simulink library "Thermal_Node"  (R2018b)
settings: Solver=ode45  StartTime=0.0  StopTime=10.0  RelTol=1e-3  EnableMultiTasking=on
settings Model: Creator=Hafner  LastModifiedBy=drhf
settings DataIOCC: LimitDataPoints=on  SaveFormat=Array  SignalLoggingSaveFormat=ModelDataLogs
settings OptimizationCC: ExpressionDepthLimit=2147483647  LifeSpan=inf
settings DebuggingCC: UnderspecifiedInitializationDetection=Classic  MergeDetectMultiDrivingBlocksExec=none  SolverPrmCheckMsg=warning  FcnCallInpInsideContextMsg=warning  StateNameClashWarn=warning  SFUnexpectedBacktrackingDiag=warning  SFNoUnconditionalDefaultTransitionDiag=warning  SFExecutionAtInitializationDiag=none
settings HardwareCC: ProdBitPerPointer=32  ProdBitPerSizeT=32  ProdBitPerPtrDiffT=32  ProdLargestAtomicFloat=None  ProdIntDivRoundTo=Undefined  ProdEndianess=Unspecified  ProdWordSize=32  ProdHWDeviceType=32-bit Generic
settings ModelReferenceCC: PropagateSignalLabelsOutOfModel=off
settings SFSimCC: SimUseLocalCustomCode=off
settings RTWCC: RTWUseLocalCustomCode=off
settings CodeAppCC: StateflowObjectComments=on
settings GRTTargetCC: TargetLangStandard=C89/C90 (ANSI)  GeneratePreprocessorConditionals=Disable all  CombineOutputUpdateFcns=off  GRTInterface=on
settings ConfigComp: CovMetricSettings=dw  CovHtmlReporting=on  CovSaveCumulativeToWorkspaceVar=on  CovSaveSingleToWorkspaceVar=on  CovExternalEMLEnable=off

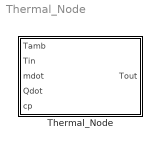
== system Thermal_Node ==
  Thermal_Node : Subsystem  mask(Thermal Capacity){UA=10, mcp=3*4182}
      mask prompts: UA "UA: thermal loss coefficient in W/K"; mcp "mcp: thermal capacity of the node in J/K"
      mask help:
      | One node model of a thermal mass based on the equation:
      |
      | mcp * dT/dt = UA*(Tamb-T) + mdot*cp_in*(Tin-T) + Qdot
      |
      | cp_in  :  heat capacity of entering fluid in J/kg/K
      | mdot  :  entering fluid massflow in kg/s
      | Qdot  :  additional thermal power added to node in W
      | Tin     :  temperature of entering massflow in °C
      | T        :  temperature of the node in °C
      mask Help: web(fullfile(path_carnot('help'),'Thermal_Node.html'),'-helpbrowser')
      mask TypeOptions UA: Losses/Gain
      mask TypeOptions mcp: nodeCapacity/Value
      mask Display: plot(-20,0,120,100,[10,70,70,10,10],[10,10,70,70,10],[70,90,90,30,10],[10,30,90,90,70],[90,70],[90,70],[50,30],[60,60],[40,40],[30,60])

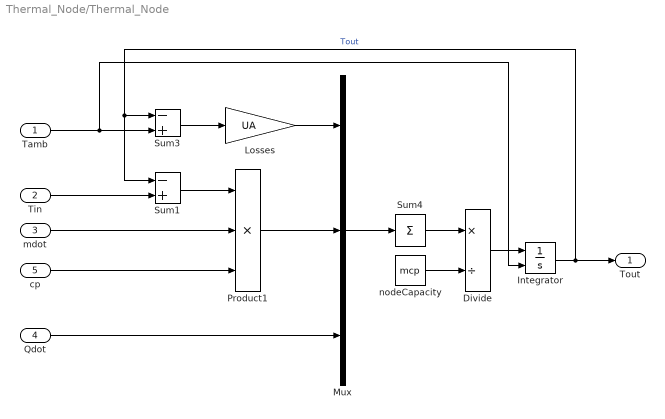
== system Thermal_Node/Thermal_Node ==
  Tamb : Inport
  Tin : Inport  Port=2
  mdot : Inport  Port=3
  Qdot : Inport  Port=4
  cp : Inport  Port=5
  Divide : Product  Inputs=*/
  Integrator : Integrator  InitialConditionSource=external  InitialCondition=40
  Losses : Gain  Gain=UA  SaturateOnIntegerOverflow=on  OutDataTypeStr=Inherit: Same as input  ParamDataTypeStr=Inherit: Same as input
  Mux : Mux  Inputs=3
  Product1 : Product  Inputs=3  SaturateOnIntegerOverflow=on  InputSameDT=on  OutDataTypeStr=Inherit: Same as first input
  Sum1 : Sum  Inputs=-+  SaturateOnIntegerOverflow=on  InputSameDT=on  OutDataTypeStr=Inherit: Same as first input
  Sum3 : Sum  Inputs=-+  SaturateOnIntegerOverflow=on  InputSameDT=on  OutDataTypeStr=Inherit: Same as first input
  Sum4 : Sum  Inputs=1  SaturateOnIntegerOverflow=on  InputSameDT=on  OutDataTypeStr=Inherit: Same as first input
  nodeCapacity : Constant  Value=mcp
  Tout : Outport  InitialOutput=40
  wires:
  Qdot/1 -> Mux/3
  Sum1/1 -> Product1/1
  Divide/1 -> Integrator/1
  cp/1 -> Product1/3
  Sum3/1 -> Losses/1
  Losses/1 -> Mux/1
  Tamb/1 -> Integrator/2, Sum3/2
  Mux/1 -> Sum4/1
  Product1/1 -> Mux/2
  Integrator/1 -> Sum3/1, Sum1/1, Tout/1  "Tout"
  Tin/1 -> Sum1/2
  mdot/1 -> Product1/2
  nodeCapacity/1 -> Divide/2
  Sum4/1 -> Divide/1
